simulink model "IntrafusalFiber"  (Simulink 7.9)
settings: Solver=ode45  StartTime=0.0  StopTime=10.0  RelTol=1e-3
undefined symbols (not defined in the file or in its folder): dfilt, fdesignblkfcn, gcbh
libraries: dsparch4 x1
settings Model: Creator=oli  LastModifiedBy=oli

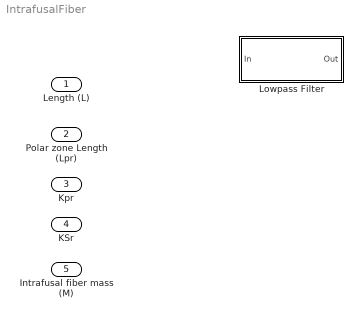
== system IntrafusalFiber ==
  Length (L) : Inport
  Polar zone Length (Lpr) : Inport  Port=2
  Kpr : Inport  Port=3
  KSr : Inport  Port=4
  Intrafusal fiber mass (M) : Inport  Port=5
  Lowpass Filter : Subsystem  DialogController=fdesignblkfcn  DialogControllerArgs=DataTag1  InitFcn=fdesignblkfcn(gcbh, {'InitFcn'});
      settings: CopyFcn=fdesignblkfcn(gcbh, {'CopyFcn'});
      mask Type: Lowpass Filter
      mask Description: Design a lowpass filter
      mask Help: helpview(mapfilelocation('dsp'), 'dsplowpassfilter');
      mask Display: disp('Lowpass')

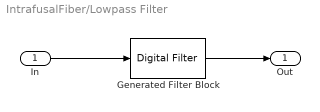
== system IntrafusalFiber/Lowpass Filter ==
  In : Inport
  Generated Filter Block : dsparch4/Digital Filter  Tag=BlockMethodSubSystem  TypePopup=FIR (all zeros)  IIRFiltStruct=Direct form II transposed  AllPoleFiltStruct=Direct form  FIRFiltStruct=Direct form  CoeffSource=Specify via dialog  NumCoeffs=[-0.00242287385232699 -0.00208324498207929 0.00677034464011864 0.016731945423489 0.0111170760810776 -0.00623114541414452 -0.00840161718602686 0.00925679761513803 0.0129828838088558 -0.010121234703279 -0.0182735187337825 0.011431962071778 0.0261758885804076 -0.012489027835323 -0.0379966231454636 0.0133889451993669 0.0581554658147299 -0.0140480435158089 -0.102724668578822 0.0144622757712384 0.317166497217695 0.485387646787325 0.317166497217695 0.0144622757712384 -0.102724668578822 -0.0140480435158089 0.0581554658147299 0.0133889451993669 -0.0379966231454636 -0.012489027835323 0.0261758885804076 0.011431962071778 -0.0182735187337825 -0.010121234703279 0.0129828838088558 0.00925679761513803 -0.00840161718602686 -0.00623114541414452 0.0111170760810776 0.016731945423489 0.00677034464011864 -0.00208324498207929 -0.00242287385232699]  DenCoeffs=[1 0.1]  BiQuadCoeffs=[1 0.3 0.4 1 0.1 0.2]  LatticeCoeffs=[0.2 0.4]  denIgnore=on  FiltPerSampPopup=One filter per frame  IC=0  ICnum=0  ICden=0  roundingMode=Floor  overflowMode=off  ScaleValues=1  scaleValueFracLength=14  stageInFracLength=15  stageOutFracLength=15  FilterSource=Specify via dialog  dfiltObjectName=dfilt.dffir([1 2 1])  InputProcessing=Columns as channels (frame based)
  Out : Outport
  wires:
  In/1 -> Generated Filter Block/1
  Generated Filter Block/1 -> Out/1
